simulink model "phdMain"  (R2023b)
settings: Solver=ode4  StartTime=0.0  StopTime=t.Data(end)  FixedStep=1e-3  RelTol=1e-3
values from neighbouring files (symbols this model uses):
  Am = T * Ac * inv(T)    [ref_model_mrac.m]
  Bm = T * Bc    [ref_model_mrac.m]
  Cm = eye(3)    [ref_model_mrac.m]
  Dm = zeros(3,1)    [ref_model_mrac.m]
undefined symbols (not defined in the file or in its folder): A_bar, AEFF, B_E, C_bar, C_T, Cd_neg, Cd_pos, DiscIntNeverNeededParam, Gamma, H, k, K, L_gain, L_STROKE, M, m3PsToLpm, P_return_Pa, P_supply_Pa, PA_Pa, PaToBar, PB_Pa, RHO, Ts, V01, V02, V_DEAD, v_mPs, W, xc_dot, xc_m
(part 3 of 3)

== matlab function phdMain/Plant/Cylinder_Dynamics/Subsystem/Subsystem/MATLAB Function ==
  data: v input; F_statik output
function F_statik = fcn(v)
Fc = 18; 
Fs = 75; 
v_s = 0.016; 
C = 100; 

F_statik = Fc + (Fs - Fc)*exp(-(1*abs(v)./v_s)^2);
F_statik = F_statik * tanh(C*v);

== matlab function phdMain/Plant/Cylinder_Dynamics/Friction_Simple ==
  data: v input; FF output
function FF = fcn(v)
eps_smooth = 0.03; 

% --- Pozitif Yön (v > 0) ---
kv_p = 20; kc_p = 15; ks_p = 82.9; tau_p = 0.016;

% --- Negatif Yön (v < 0) ---
kv_n = 35; kc_n = 22; ks_n = 75.17; tau_n = 0.016;

% Yumuşatılmış yön fonksiyonu (sign yerine tanh)
% Bu fonksiyon -1 ile 1 arasında yumuşak bir geçiş sağlar
smooth_sign = tanh(v ./ eps_smooth);

% Asimetrik katsayı vektörleri oluşturma
% Hızın yönüne göre katsayıları seçiyoruz
kv = (v >= 0)*kv_p + (v < 0)*kv_n;
kc = (v >= 0)*kc_p + (v < 0)*kc_n;
ks = (v >= 0)*ks_p + (v < 0)*ks_n;
tau = (v >= 0)*tau_p + (v < 0)*tau_n;

% --- Sürtünme Kuvveti Hesaplama ---
% F_viscous + F_coulomb + F_stribeck
FF = (kv .* v) + (kc .* smooth_sign) + (ks .* smooth_sign .* exp(-abs(v./tau)));
